simulink subsystem "Rigid"  (R2025b)
settings: Solver=VariableStepAuto  StartTime=0.0  StopTime=10.0  RelTol=1e-3
settings Model: Creator=The MathWorks, Inc.  LastModifiedBy=The MathWorks, Inc.
settings RTWCC: GPUComputeCapability=3.5

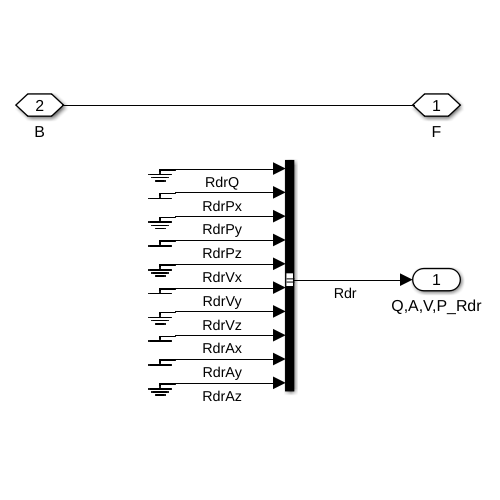
[thumbnail: Simulink's stored preview of the top-level diagram]
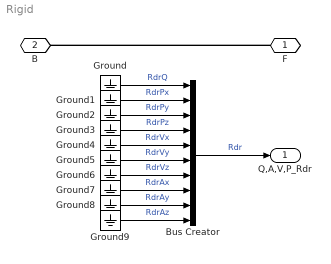
== system Rigid ==
  Bus Creator : BusCreator  Inputs=10
  Ground{,1..9} (10 alike) : Ground
  F : PMIOPort  Side=Right
  B : PMIOPort  Port=2  Side=Left
  Q,A,V,P_Rdr : Outport
  wires:
  Ground5/1 -> Bus Creator/6  "RdrVy"
  Ground6/1 -> Bus Creator/7  "RdrVz"
  Ground4/1 -> Bus Creator/5  "RdrVx"
  Ground3/1 -> Bus Creator/4  "RdrPz"
  Ground2/1 -> Bus Creator/3  "RdrPy"
  Bus Creator/1 -> Q,A,V,P_Rdr/1  "Rdr"
  Ground/1 -> Bus Creator/1  "RdrQ"
  Ground9/1 -> Bus Creator/10  "RdrAz"
  Ground1/1 -> Bus Creator/2  "RdrPx"
  Ground8/1 -> Bus Creator/9  "RdrAy"
  Ground7/1 -> Bus Creator/8  "RdrAx"
  connections:
  F/RConn1 -- B/RConn1
